simulink model "linearizedModel"  (R2019b)
settings: Solver=VariableStepAuto  StartTime=0.0  StopTime=10.0  RelTol=1e-3
values from neighbouring files (symbols this model uses):
  A_rot = zeros(6, 6)    [linearModel.m]
  A_trans = zeros(6, 6)    [linearModel.m]
  B_rot = [param.drone.I^-1 ... (first row only)    [linearModel.m]
  B_trans = [0                param.env.g*sin(param.sp.psi0)  param.env.g*cos(param.sp.psi0)   0 ... (first row only)    [linearModel.m]
  C_rot = eye(6)    [linearModel.m]
  C_trans = eye(6)    [linearModel.m]
  D_rot = zeros(6, 3)    [linearModel.m]
  D_trans = zeros(6, 4)    [linearModel.m]
  param = struct()    [parameters.m]
undefined symbols (not defined in the file or in its folder): K_rot
settings Model: Creator=emiel  LastModifiedBy=emiel

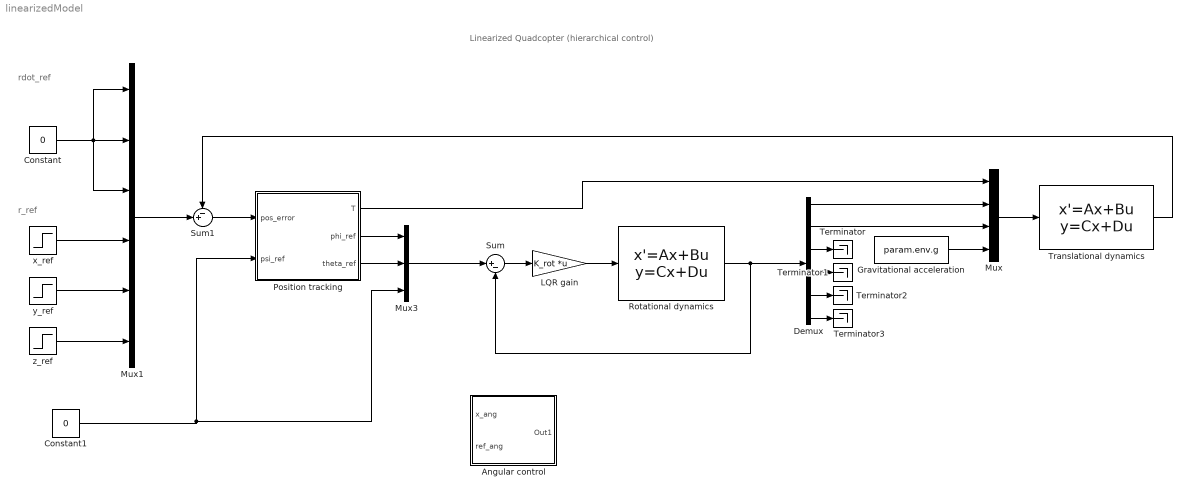
== system linearizedModel ==
  note: rdot_ref
  note: r_ref
  note: Linearized Quadcopter (hierarchical control)
  Angular control : Subsystem
  Constant : Constant  Value=0
  Constant1 : Constant  Value=0
  Demux : Demux  Outputs=6
  Gravitational acceleration : Constant  Value=param.env.g
  LQR gain : Gain  Gain=K_rot  Multiplication=Matrix(K*u) (u vector)
      settings: AttributesFormatString=%<Gain>
  Mux : Mux
  Mux1 : Mux  Inputs=6
  Mux3 : Mux  Inputs=3
  Position tracking : Subsystem
  Rotational dynamics : StateSpace  A=A_rot  B=B_rot  C=C_rot  D=D_rot  InitialCondition=0
  Sum : Sum  Inputs=|+-
  Sum1 : Sum  Inputs=-+|
  Terminator{,1..3} (4 alike) : Terminator
  Translational dynamics : StateSpace  A=A_trans  B=B_trans  C=C_trans  D=D_trans  InitialCondition=0
  x_ref : Step  After=5  SampleTime=0
  y_ref : Step  After=2  SampleTime=0
  z_ref : Step  After=3  SampleTime=0
  wires:
  Rotational dynamics/1 -> Demux/1, Sum/2
  Sum/1 -> LQR gain/1
  LQR gain/1 -> Rotational dynamics/1
  Demux/1 -> Mux/2
  Demux/2 -> Mux/3
  Gravitational acceleration/1 -> Mux/4
  Mux/1 -> Translational dynamics/1
  Sum1/1 -> Position tracking/1(pos_error)
  Demux/3 -> Terminator/1
  Demux/4 -> Terminator1/1
  Demux/5 -> Terminator2/1
  Demux/6 -> Terminator3/1
  Position tracking/1(T) -> Mux/1
  x_ref/1 -> Mux1/4
  y_ref/1 -> Mux1/5
  z_ref/1 -> Mux1/6
  Constant/1 -> Mux1/3, Mux1/1, Mux1/2
  Mux1/1 -> Sum1/2
  Translational dynamics/1 -> Sum1/1
  Constant1/1 -> Mux3/3, Position tracking/2(psi_ref)
  Position tracking/2(phi_ref) -> Mux3/1
  Position tracking/3(theta_ref) -> Mux3/2
  Mux3/1 -> Sum/1

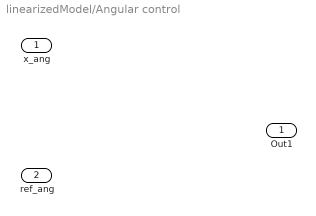
== system linearizedModel/Angular control ==
  x_ang : Inport
  ref_ang : Inport  Port=2
  Out1 : Outport

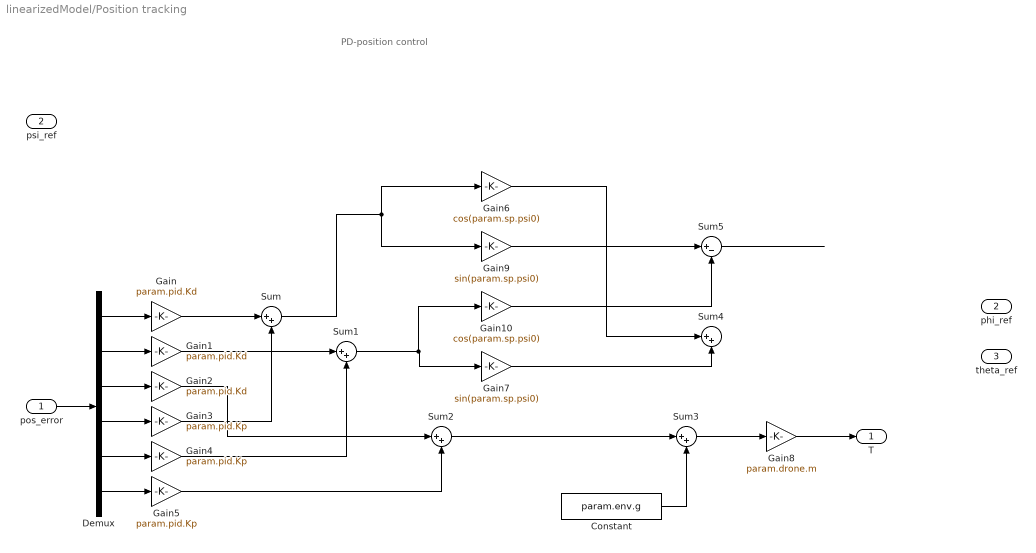
== system linearizedModel/Position tracking ==
  note: PD-position control
  pos_error : Inport
  psi_ref : Inport  Port=2
  Constant : Constant  Value=param.env.g
  Demux : Demux  Outputs=6
  Gain : Gain  Gain=param.pid.Kd
  Gain1 : Gain  Gain=param.pid.Kd
  Gain10 : Gain  Gain=cos(param.sp.psi0)
      settings: AttributesFormatString=%<Gain>
  Gain2 : Gain  Gain=param.pid.Kd
  Gain3 : Gain  Gain=param.pid.Kp
  Gain4 : Gain  Gain=param.pid.Kp
  Gain5 : Gain  Gain=param.pid.Kp
  Gain6 : Gain  Gain=cos(param.sp.psi0)
      settings: AttributesFormatString=%<Gain>
  Gain7 : Gain  Gain=sin(param.sp.psi0)
      settings: AttributesFormatString=%<Gain>
  Gain8 : Gain  Gain=param.drone.m
      settings: AttributesFormatString=%<Gain>
  Gain9 : Gain  Gain=sin(param.sp.psi0)
      settings: AttributesFormatString=%<Gain>
  Sum{,1..4} (5 alike) : Sum  Inputs=|++
  Sum5 : Sum  Inputs=|+-
  T : Outport
  phi_ref : Outport  Port=2
  theta_ref : Outport  Port=3
  wires:
  pos_error/1 -> Demux/1
  Demux/1 -> Gain/1
  Demux/2 -> Gain1/1
  Demux/3 -> Gain2/1
  Demux/4 -> Gain3/1
  Demux/5 -> Gain4/1
  Demux/6 -> Gain5/1
  Gain/1 -> Sum/1
  Gain3/1 -> Sum/2
  Gain1/1 -> Sum1/1
  Gain4/1 -> Sum1/2
  Gain2/1 -> Sum2/1
  Gain5/1 -> Sum2/2
  Sum/1 -> Gain9/1, Gain6/1
  Sum1/1 -> Gain10/1, Gain7/1
  Sum2/1 -> Sum3/1
  Constant/1 -> Sum3/2
  Sum3/1 -> Gain8/1
  Gain8/1 -> T/1
  Gain9/1 -> Sum5/1
  Gain10/1 -> Sum5/2
  Gain6/1 -> Sum4/1
  Gain7/1 -> Sum4/2
  Sum5/1 -> ?
